simulink model "pulse_heating_official_spine_v04"  (R2025b)
settings: Solver=VariableStepAuto  StartTime=0.0  StopTime=0.25  RelTol=1e-3
PreLoadFcn:
  | addpath('C:\Users\ADMIN\Documents\MATLAB\Examples\R2025b\simscapeelectrical\BatteryThermalManagementExample');
  | addpath('C:\Users\ADMIN\Documents\MATLAB\Examples\R2025b\mcb\SIUnitsExample');
  | addpath('C:\Users\ADMIN\Documents\MATLAB\Examples\R2025b\simscapeelectrical\PMSMDriveThermalExample');
  | load_system('PMSMDriveThermal');
  | set_param('PMSMDriveThermal','SimscapeLogType','none','SimscapeLogSimulationStatistics','off');
  | set_param('PMSMDriveThermal','Dirty','off');
InitFcn:
  | % === M4-02A: Clean parameter matching (MO theory PI) ===
  | addpath('C:\Users\ADMIN\Documents\MATLAB\Examples\R2025b\simscapeelectrical\BatteryThermalManagementExample');
  | addpath('C:\Users\ADMIN\Documents\MATLAB\Examples\R2025b\mcb\SIUnitsExample');
  | addpath('C:\Users\ADMIN\Documents\MATLAB\Examples\R2025b\simscapeelectrical\PMSMDriveThermalExample');
  | load_system('PMSMDriveThermal');
  | PMSMDriveThermalData;
  | mcb_pmsm_foc_qep_f28379d_SIUnit_data;
  | clearvars('all');
  | 
  | % --- Construct clean pmsm struct from PMSMDriveThermal ---
  | pmsm = struct();
  | pmsm.Rs = Rs; pmsm.Ld = Ld; pmsm.Lq = Lq; pmsm.p = N; pmsm.FluxPM = PM;
  | pmsm.J = J; pmsm.B = 2.6369e-6; pmsm.I_rated = Imax;
  | pmsm.Ke = PM*N; pmsm.Kt = 1.5*N*PM; pmsm.N_max = 60*fnom/N;
  | pmsm.PositionOffset = 0; pmsm.QEPSlits = 1000;
  | 
  | inverter.V_dc = 70; dataType = 'double';
  | pmsm.N_base = inverter.V_dc / (sqrt(3)*PM*N*2*pi/60);
  | pmsm.T_rated = 1.5*N*PM*Imax;
  | 
  | % --- Timing (PMSMDriveThermal semantics) ---
  | Ts = 2e-6; fsw = 2e3; fc = fsw*10; Tsc = 1/fc;
  | T_pwm = 1/fsw; PWM_frequency = fsw; Ts_simulink = Tsc;
  | Ts_motor = Tsc; Ts_speed = 10*Tsc; Ts_inverter = Tsc;
  | 
  | % --- PI gains via mcb.calcFOCGains (MO theory) ---
  | motor = pmsm; motor.Rs = pmsm.Rs + inverter.R_board;
  | PI_params = mcb.calcFOCGains(motor, Tsc, Ts_speed, SpdLPFltCoeff=0.01);
  | PI_params.delay_Currents = int32(1);
  | PI_params.delay_Position = int32(1);
  | 
  | BatteryThermalManagementInitialization;
  | ambient = 263.15; coolantTemp = 263.15;
  | cellT_ini = ambient*ones(1,Ns*Np); cellT_ini4 = ambient*ones(1,Ns4*Np4);
  | Ns_total = 3*Ns + Ns4; Np_total = Np;
  | R_pack = Ns_total * R0_mat(3,2) / Np_total;
  | I_base_A = AH * Np_total; V_pack_nom = Ns_total * 3.3;
  | 
  | % === M4-01 generalized Reference / Platform contract ===
  | % Values are traceable engineering/platform defaults, not device ratings.
  | ReferenceConfig_ID = 'M4-01-REF-PLATFORM-v02';
  | ReferenceConfig_Source = 'OFFICIAL+ENGINEERING_DEFAULT';
  | ReferenceConfig_Scope = 'generalized_system_integration';
  | HVPath_R = 0.01;
  | DCLink_C = 470e-6;
  | DCLink_V0 = 0;
  | RMS_Window_s = 20/fsw;
  | IGBT_Ron_ref = 1e-3;
  | IGBT_Vf_ref = 1.2;
  | 
  | % Encoder/reference topology provides the static mechanical boundary.
  | OpenLoop_Vabc_Scale = 1;
model workspace (MAT data in the model file):
  control_status_v4d2_partial_duty_code = 6
  diagnostic_frequency_Hz = 50
  drive_status_v4d2_partial_current_code = 6
  kpi_status_v4d2_partial_numeric_code = 6
  kpi_value_unknown = nan
  limit_factor_unknown_code = 99
  limit_margin_unknown_value = nan
  limit_status_v4c_code = 5
  pulse_command_status_code = 6
  pulse_duty_percent = 50
  pulse_id_amplitude_A = 40
  pulse_iq_amplitude_A = 0
  pulse_mode_code = 4
  pulse_phase_delay_s = 0
undefined symbols (not defined in the file or in its folder): DiscIntNeverNeededParam, f_losses, Flowrate_vec, Isc_losses, losses_oc, losses_sc, N, PM, Rs
libraries: fl_lib x38, nesl_utility x35, ee_lib x12, mcbcontrolslib x5, mcbeeMathTransformLib x3, slpidlib x2, mcbhdlpositiondecoderlib x1, eePwmGeneratorTwoLevel x1
(part 4 of 4)

== system pulse_heating_official_spine_v04/PMSMDriveThermal_Inverter_And_Motor/Thermal model/Sensing Temperature WiA ==
  PS-Simulink Converter : nesl_utility/PS-Simulink Converter  PhysicalDomain=network_engine_domain  SubClassName=ps_output  LeftPortType=input  RightPortType=output  PseudoPeriodic=off  Frequencies=[]  VectorFormat=1-D array  Unit=degC  AffineConversion=on
  Temperature Sensor : fl_lib/Thermal/Thermal Sensors/Temperature Sensor  temperature_measure=foundation.enum.MeasurementReference.difference
  ThRef : fl_lib/Thermal/Thermal Elements/Thermal Reference
  H : PMIOPort  Side=Left
  tag scope: TA=global
  wires:
  PS-Simulink Converter/1 -> [TA]
  connections:
  Temperature Sensor/RConn2 -- PS-Simulink Converter/LConn1
  ThRef/LConn1 -- Temperature Sensor/RConn1
  H/RConn1 -- Temperature Sensor/LConn1

== system pulse_heating_official_spine_v04/PMSMDriveThermal_Inverter_And_Motor/Thermal model/Sensing Temperature WiB ==
  PS-Simulink Converter : nesl_utility/PS-Simulink Converter  PhysicalDomain=network_engine_domain  SubClassName=ps_output  LeftPortType=input  RightPortType=output  PseudoPeriodic=off  Frequencies=[]  VectorFormat=1-D array  Unit=degC  AffineConversion=on
  Temperature Sensor : fl_lib/Thermal/Thermal Sensors/Temperature Sensor  temperature_measure=foundation.enum.MeasurementReference.difference
  ThRef : fl_lib/Thermal/Thermal Elements/Thermal Reference
  H : PMIOPort  Side=Left
  tag scope: TB=global
  wires:
  PS-Simulink Converter/1 -> [TB]
  connections:
  H/RConn1 -- Temperature Sensor/LConn1
  ThRef/LConn1 -- Temperature Sensor/RConn1
  Temperature Sensor/RConn2 -- PS-Simulink Converter/LConn1

== system pulse_heating_official_spine_v04/PMSMDriveThermal_Inverter_And_Motor/Thermal model/Sensing Temperature WiC ==
  PS-Simulink Converter : nesl_utility/PS-Simulink Converter  PhysicalDomain=network_engine_domain  SubClassName=ps_output  LeftPortType=input  RightPortType=output  PseudoPeriodic=off  Frequencies=[]  VectorFormat=1-D array  Unit=degC  AffineConversion=on
  Temperature Sensor : fl_lib/Thermal/Thermal Sensors/Temperature Sensor  temperature_measure=foundation.enum.MeasurementReference.difference
  ThRef : fl_lib/Thermal/Thermal Elements/Thermal Reference
  H : PMIOPort  Side=Left
  tag scope: TC=global
  wires:
  PS-Simulink Converter/1 -> [TC]
  connections:
  Temperature Sensor/RConn2 -- PS-Simulink Converter/LConn1
  ThRef/LConn1 -- Temperature Sensor/RConn1
  H/RConn1 -- Temperature Sensor/LConn1

== system pulse_heating_official_spine_v04/BatteryThermalManagement_BatteryPack/Coolant_control/FlwR estimation/FlwR=f(cell_deltaT) ==
  Pack max T : Inport
  Pack min T : Inport  Port=2
  limit FlwR : Inport  Port=3
  MinMax4 : MinMax  Inputs=2  ZeroCross=off
  Multiply : Gain  Gain=0.1
  Subtract : Sum  Inputs=+-
  FlwR : Outport
  wires:
  Pack min T/1 -> Subtract/2
  MinMax4/1 -> FlwR/1
  Pack max T/1 -> Subtract/1
  Multiply/1 -> MinMax4/1
  limit FlwR/1 -> MinMax4/2
  Subtract/1 -> Multiply/1

== system pulse_heating_official_spine_v04/BatteryThermalManagement_BatteryPack/Coolant_control/FlwR estimation/FlwR=f(packT-ambientT) ==
  Pack max T : Inport
  FlwR limit : Inport  Port=2
  Ambient T : Inport  Port=3
  MinMax1 : MinMax  Inputs=2  ZeroCross=off
  Multiply1 : Gain  Gain=0.1
  Subtract1 : Sum  Inputs=+-
  FlwR : Outport
  wires:
  Ambient T/1 -> Subtract1/2
  MinMax1/1 -> FlwR/1
  Pack max T/1 -> Subtract1/1
  FlwR limit/1 -> MinMax1/1
  Multiply1/1 -> MinMax1/2
  Subtract1/1 -> Multiply1/1

== system pulse_heating_official_spine_v04/BatteryThermalManagement_BatteryPack/Coolant_control/Subsystem1/Flowrate-value ==
  FlwR : Inport
  Flowrate vector : Inport  Port=2
  MinMax6 : MinMax  Function=max  ZeroCross=off
  Product : Product
  Flowrate : Outport
  wires:
  Flowrate vector/1 -> MinMax6/1
  Product/1 -> Flowrate/1
  FlwR/1 -> Product/1
  MinMax6/1 -> Product/2

== system pulse_heating_official_spine_v04/BatteryThermalManagement_BatteryPack/Coolant_control/Subsystem1/FlwR limits ==
  FlwR : Inport
  MinMax5 : MinMax  Function=max  Inputs=2  ZeroCross=off
  MinMax7 : MinMax  Inputs=2  ZeroCross=off
  max value : Constant
  min value : Constant  Value=0.001
  FlwR_out : Outport
  wires:
  MinMax7/1 -> FlwR_out/1
  MinMax5/1 -> MinMax7/2
  FlwR/1 -> MinMax5/1
  max value/1 -> MinMax7/1
  min value/1 -> MinMax5/2

== system pulse_heating_official_spine_v04/BatteryThermalManagement_BatteryPack/Coolant_control/Subsystem1/Step generator ==
  frac : Inport
  step size : Inport  Port=2
  Max5 : MinMax  Function=max  Inputs=2  ZeroCross=off
  Minus4 : Sum  Inputs=+-
  Mod : Math  Operator=mod
  step output : Outport
  wires:
  frac/1 -> Mod/1, Minus4/1
  Max5/1 -> step output/1
  step size/1 -> Mod/2, Max5/2
  Mod/1 -> Minus4/2
  Minus4/1 -> Max5/1

== system pulse_heating_official_spine_v04/MCB_SIUnits_FOC_Controller/Control_System/Closed Loop Control/Current_Controllers ==
  Id : Inport
  Iq : Inport  Port=2
  Ida_ref : Inport  Port=3
  DQ Limiter : mcbcontrolslib/DQ Limiter  satMethodInputType=Specify via dialog  satMethodSelected=D-Q equivalence  satLimitInputType=Specify via dialog  Vmax=inverter.V_dc/sqrt(3) *0.95
  Demux : Demux  Outputs=2
  Mux : Mux
  PI_Controller_Id : Subsystem
  PI_Controller_Iq : Subsystem
  Terminator : Terminator
  Vd_ref : Outport  VectorParamsAs1DForOutWhenUnconnected=off
  Vq_ref : Outport  Port=2  VectorParamsAs1DForOutWhenUnconnected=off
  Idq : Outport  Port=3  VectorParamsAs1DForOutWhenUnconnected=off
  wires:
  DQ Limiter/3 -> Terminator/1
  DQ Limiter/1 -> Vd_ref/1
  DQ Limiter/2 -> Vq_ref/1
  PI_Controller_Iq/1(V_ref) -> DQ Limiter/2
  PI_Controller_Id/1(V_ref) -> DQ Limiter/1
  Mux/1 -> Idq/1
  Ida_ref/1 -> Demux/1
  Demux/2 -> PI_Controller_Iq/1(I_ref), Mux/3  "Iq_Ref"
  Demux/1 -> PI_Controller_Id/1(I_ref), Mux/1  "Id_Ref"
  Id/1 -> PI_Controller_Id/2(I_fb), Mux/2  "Id_fb"
  Iq/1 -> PI_Controller_Iq/2(I_fb), Mux/4  "Iq_fb"

== system pulse_heating_official_spine_v04/MCB_SIUnits_FOC_Controller/Control_System/Closed Loop Control/SVPWM ==
  Va : Inport
  Vb : Inport  Port=2
  Constant : Constant  Value=0.5  OutDataTypeStr=dataType  SampleTime=-1
  Mux1 : Mux  Inputs=3
  Normalize [-0.5 to 0.5] : Gain  Gain=1/ (2 * inverter.V_dc / sqrt(3))  RndMeth=Simplest  OutDataTypeStr=Inherit: Same as input
  Space Vector Generator : mcbcontrolslib/PWM Reference Generator  inSignal=Valphabeta  modType=SVM: space vector modulation
  Sum : Sum  Inputs=|++
  Duty_abc : Outport
  wires:
  Sum/1 -> Duty_abc/1
  Vb/1 -> Space Vector Generator/2
  Space Vector Generator/2 -> Mux1/2
  Space Vector Generator/3 -> Mux1/3
  Constant/1 -> Sum/2
  Space Vector Generator/1 -> Mux1/1
  Va/1 -> Space Vector Generator/1
  Normalize [-0.5 to 0.5]/1 -> Sum/1
  Mux1/1 -> Normalize [-0.5 to 0.5]/1

== system pulse_heating_official_spine_v04/MCB_SIUnits_FOC_Controller/Control_System/Open Loop Start-Up/Convert to Duty Cycles ==
  In : Inport
  Constant : Constant  Value=0.5  OutDataTypeStr=dataType  SampleTime=-1
  Normalize : Gain  Gain=1/2  RndMeth=Simplest  OutDataTypeStr=Inherit: Same as input
  Sum1 : Sum  Inputs=|++
  Out : Outport
  wires:
  Sum1/1 -> Out/1
  In/1 -> Normalize/1
  Constant/1 -> Sum1/2
  Normalize/1 -> Sum1/1

== system pulse_heating_official_spine_v04/MCB_SIUnits_FOC_Controller/Control_System/Open Loop Start-Up/Ramp Generator ==
  Ramp_Time : Inport
  Enable : Inport  Port=2
  Divide : Product  Inputs=*/  RndMeth=Simplest  OutDataTypeStr=Inherit: Same as first input
  NOT : Logic  Operator=NOT  IconShape=distinctive  AllPortsSameDT=off  OutDataTypeStr=boolean
  One : Constant  OutDataTypeStr=dataType  SampleTime=-1
  Ramp Generator : DiscreteIntegrator  IntegratorMethod=Accumulation: Forward Euler  gainval=1  ExternalReset=sampled level  SampleTime=-1  OutDataTypeStr=dataType  RndMeth=Simplest  LimitOutput=on  UpperSaturationLimit=1  LowerSaturationLimit=0  ICPrevOutput=DiscIntNeverNeededParam  ICPrevScaledInput=DiscIntNeverNeededParam
  Sample_Time : Gain  Gain=Tsc  RndMeth=Simplest  OutDataTypeStr=Inherit: Same as input
  Ramp : Outport
  wires:
  NOT/1 -> Ramp Generator/2
  Enable/1 -> NOT/1
  Ramp_Time/1 -> Divide/2
  One/1 -> Divide/1
  Sample_Time/1 -> Ramp Generator/1
  Ramp Generator/1 -> Ramp/1  "Eps"
  Divide/1 -> Sample_Time/1

== system pulse_heating_official_spine_v04/MCB_SIUnits_FOC_Controller/Control_System/Closed Loop Control/Current_Controllers/PI_Controller_Id ==
  I_ref : Inport
  I_fb : Inport  Port=2
  Data Store Read1 : DataStoreRead  DataStoreName=Enable  IndexOptions=Index vector (dialog)  Indices=1  OutputSizes=1
  Discrete PI Controller with anti-windup & reset : slpidlib/PID Controller  Controller=PI  Form=Parallel  TimeDomain=Discrete-time  UseExternalTs=off  SampleTime=-1  IntegratorMethod=Forward Euler  FilterMethod=Forward Euler  ControllerParametersSource=external  P=1  I=1  UseKiTs=on  D=0  UseExternalDerivativeSource=off  N=100  UseFilter=on  TunerSelectOption=Transfer Function Based (PID Tuner App)  InitialConditionSource=external  InitialConditionForIntegrator=0  InitialConditionForFilter=0  DifferentiatorICPrevScaledInput=0  ExternalReset=level  TrackingMode=off  Kt=1  LimitOutput=on  SatLimitsSource=internal  UpperSaturationLimit=inverter.V_dc/sqrt(3)  LowerSaturationLimit=-inverter.V_dc/sqrt(3)  LinearizeAsGain=on  AntiWindupMode=clamping  Kb=1  LimitIntegrator=off  UpperIntegratorSaturationLimit=inf  LowerIntegratorSaturationLimit=-inf  RndMeth=Simplest  POutMin=[]  POutMax=[]  IOutMin=[]  IOutMax=[]  DOutMin=[]  DOutMax=[]  NOutMin=[]  NOutMax=[]  SumOutMin=[]  SumOutMax=[]  SaturationOutDataTypeStr=Inherit: Inherit via back propagation  SaturationOutMin=[]  SaturationOutMax=[]  PParamMin=[]  PParamMax=[]  IParamMin=[]  IParamMax=[]  DParamMin=[]  DParamMax=[]  NParamMin=[]  NParamMax=[]  KbParamMin=[]  KbParamMax=[]  KtParamMin=[]  KtParamMax=[]  KbOutMin=[]  KbOutMax=[]  KtOutMin=[]  KtOutMax=[]  IntegratorOutMin=[]  IntegratorOutMax=[]  FilterOutMin=[]  FilterOutMax=[]  SumI1OutMin=[]  SumI1OutMax=[]  SumI2OutMin=[]  SumI2OutMax=[]  SumI3OutMin=[]  SumI3OutMax=[]  SumI4OutMin=[]  SumI4OutMax=[]  SumDOutMin=[]  SumDOutMax=[]  DifferentiatorOutMin=[]  DifferentiatorOutMax=[]  FilterDiffOutCoefMin=[]  FilterDiffOutCoefMax=[]  ReciprocalOutMin=[]  ReciprocalOutMax=[]  SumDenOutMin=[]  SumDenOutMax=[]  SumNumOutMin=[]  SumNumOutMax=[]  DivideOutMin=[]  DivideOutMax=[]  UdiffTsProdOutMin=[]  UdiffTsProdOutMax=[]  NTsProdOutMin=[]  NTsProdOutMax=[]  UintegralTsProdOutMin=[]  UintegralTsProdOutMax=[]  UngainTsProdOutMin=[]  UngainTsProdOutMax=[]  ClampingZeroOutDataTypeStr=Inherit: Inherit via back propagation  ClampingZeroOutMin=[]  ClampingZeroOutMax=[]  FilterDenConstantOutDataTypeStr=Inherit: Inherit via back propagation  FilterDenConstantOutMin=[]  FilterDenConstantOutMax=[]  PCopyOutDataTypeStr=Inherit: Inherit via back propagation  PCopyOutMin=[]  PCopyOutMax=[]  NCopyOutDataTypeStr=Inherit: Inherit via back propagation  NCopyOutMin=[]  NCopyOutMax=[]  IntegratorContinuousStateAttributes=''  IntegratorStateMustResolveToSignalObject=off  IntegratorRTWStateStorageClass=Auto  FilterContinuousStateAttributes=''  FilterStateMustResolveToSignalObject=off  FilterRTWStateStorageClass=Auto  ParallelPVariant=ExternalParameters  IdealPVariant=Disabled  IVariant=ExternalParameters  DVariant=Disabled  IntegratorVariant=Discrete  SatVariant=Enabled  AWVariant=DiscClampingParallel  PCopyVariant=Disabled  TRVariant=Disabled  FdbkBlocksVariant=Forward  IdealPFdbkVariant=Disabled  SatFdbkVariant=Disabled  DerivativeFilterVariant=Disabled  NVariant=Disabled  NCopyVariant=Disabled_SignalSpec  FilterICVariant=Disabled  IntegratorICVariant=ExternalICs  ExternalResetVariant=ExternalReset  TRSumVariant=Passthrough  SumFdbkVariant=Disabled  SumVariant=Sum_PI  TsampFilterVariant=InternalTs  TsampNgainVariant=Passthrough  TsampIntegralVariant=Disabled_SignalSpec  ExternalSaturationOutDataTypeStr=Inherit: Same as second input  DerivativeSourceVariant=Disabled  PreIntVariant=InternalPreInt
      settings: LibrarySourceBlock=mcbcontrolslib/PI Controller
  Ki : Constant  Value=PI_params.Ki_i * Tsc  OutDataTypeStr=dataType  SampleTime=-1
  Ki1 : Constant  Value=0  OutDataTypeStr=dataType  SampleTime=-1
  Kp : Constant  Value=PI_params.Kp_i  OutDataTypeStr=dataType  SampleTime=-1
  Logical Operator : Logic  Operator=NOT  IconShape=distinctive  AllPortsSameDT=off  OutDataTypeStr=boolean
  Sum : Sum  Inputs=|+-  OutDataTypeStr=Inherit: Same as first input
  V_ref : Outport  VectorParamsAs1DForOutWhenUnconnected=off
  wires:
  Ki1/1 -> Discrete PI Controller with anti-windup & reset/5
  Logical Operator/1 -> Discrete PI Controller with anti-windup & reset/4
  Ki/1 -> Discrete PI Controller with anti-windup & reset/3
  Kp/1 -> Discrete PI Controller with anti-windup & reset/2
  Sum/1 -> Discrete PI Controller with anti-windup & reset/1
  Discrete PI Controller with anti-windup & reset/1 -> V_ref/1
  Data Store Read1/1 -> Logical Operator/1
  I_fb/1 -> Sum/2
  I_ref/1 -> Sum/1

== system pulse_heating_official_spine_v04/MCB_SIUnits_FOC_Controller/Control_System/Closed Loop Control/Current_Controllers/PI_Controller_Iq ==
  I_ref : Inport
  I_fb : Inport  Port=2
  Data Store Read1 : DataStoreRead  DataStoreName=Enable  IndexOptions=Index vector (dialog)  Indices=1  OutputSizes=1
  Discrete PI Controller with anti-windup & reset : slpidlib/PID Controller  Controller=PI  Form=Parallel  TimeDomain=Discrete-time  UseExternalTs=off  SampleTime=-1  IntegratorMethod=Forward Euler  FilterMethod=Forward Euler  ControllerParametersSource=external  P=1  I=1  UseKiTs=on  D=0  UseExternalDerivativeSource=off  N=100  UseFilter=on  TunerSelectOption=Transfer Function Based (PID Tuner App)  InitialConditionSource=external  InitialConditionForIntegrator=0  InitialConditionForFilter=0  DifferentiatorICPrevScaledInput=0  ExternalReset=level  TrackingMode=off  Kt=1  LimitOutput=on  SatLimitsSource=internal  UpperSaturationLimit=inverter.V_dc/sqrt(3)  LowerSaturationLimit=-inverter.V_dc/sqrt(3)  LinearizeAsGain=on  AntiWindupMode=clamping  Kb=1  LimitIntegrator=off  UpperIntegratorSaturationLimit=inf  LowerIntegratorSaturationLimit=-inf  RndMeth=Simplest  POutMin=[]  POutMax=[]  IOutMin=[]  IOutMax=[]  DOutMin=[]  DOutMax=[]  NOutMin=[]  NOutMax=[]  SumOutMin=[]  SumOutMax=[]  SaturationOutDataTypeStr=Inherit: Inherit via back propagation  SaturationOutMin=[]  SaturationOutMax=[]  PParamMin=[]  PParamMax=[]  IParamMin=[]  IParamMax=[]  DParamMin=[]  DParamMax=[]  NParamMin=[]  NParamMax=[]  KbParamMin=[]  KbParamMax=[]  KtParamMin=[]  KtParamMax=[]  KbOutMin=[]  KbOutMax=[]  KtOutMin=[]  KtOutMax=[]  IntegratorOutMin=[]  IntegratorOutMax=[]  FilterOutMin=[]  FilterOutMax=[]  SumI1OutMin=[]  SumI1OutMax=[]  SumI2OutMin=[]  SumI2OutMax=[]  SumI3OutMin=[]  SumI3OutMax=[]  SumI4OutMin=[]  SumI4OutMax=[]  SumDOutMin=[]  SumDOutMax=[]  DifferentiatorOutMin=[]  DifferentiatorOutMax=[]  FilterDiffOutCoefMin=[]  FilterDiffOutCoefMax=[]  ReciprocalOutMin=[]  ReciprocalOutMax=[]  SumDenOutMin=[]  SumDenOutMax=[]  SumNumOutMin=[]  SumNumOutMax=[]  DivideOutMin=[]  DivideOutMax=[]  UdiffTsProdOutMin=[]  UdiffTsProdOutMax=[]  NTsProdOutMin=[]  NTsProdOutMax=[]  UintegralTsProdOutMin=[]  UintegralTsProdOutMax=[]  UngainTsProdOutMin=[]  UngainTsProdOutMax=[]  ClampingZeroOutDataTypeStr=Inherit: Inherit via back propagation  ClampingZeroOutMin=[]  ClampingZeroOutMax=[]  FilterDenConstantOutDataTypeStr=Inherit: Inherit via back propagation  FilterDenConstantOutMin=[]  FilterDenConstantOutMax=[]  PCopyOutDataTypeStr=Inherit: Inherit via back propagation  PCopyOutMin=[]  PCopyOutMax=[]  NCopyOutDataTypeStr=Inherit: Inherit via back propagation  NCopyOutMin=[]  NCopyOutMax=[]  IntegratorContinuousStateAttributes=''  IntegratorStateMustResolveToSignalObject=off  IntegratorRTWStateStorageClass=Auto  FilterContinuousStateAttributes=''  FilterStateMustResolveToSignalObject=off  FilterRTWStateStorageClass=Auto  ParallelPVariant=ExternalParameters  IdealPVariant=Disabled  IVariant=ExternalParameters  DVariant=Disabled  IntegratorVariant=Discrete  SatVariant=Enabled  AWVariant=DiscClampingParallel  PCopyVariant=Disabled  TRVariant=Disabled  FdbkBlocksVariant=Forward  IdealPFdbkVariant=Disabled  SatFdbkVariant=Disabled  DerivativeFilterVariant=Disabled  NVariant=Disabled  NCopyVariant=Disabled_SignalSpec  FilterICVariant=Disabled  IntegratorICVariant=ExternalICs  ExternalResetVariant=ExternalReset  TRSumVariant=Passthrough  SumFdbkVariant=Disabled  SumVariant=Sum_PI  TsampFilterVariant=InternalTs  TsampNgainVariant=Passthrough  TsampIntegralVariant=Disabled_SignalSpec  ExternalSaturationOutDataTypeStr=Inherit: Same as second input  DerivativeSourceVariant=Disabled  PreIntVariant=InternalPreInt
      settings: LibrarySourceBlock=mcbcontrolslib/PI Controller
  Ki : Constant  Value=PI_params.Ki_i * Tsc  OutDataTypeStr=dataType  SampleTime=-1
  Kp : Constant  Value=PI_params.Kp_i  OutDataTypeStr=dataType  SampleTime=-1
  Kp1 : Constant  Value=0  OutDataTypeStr=dataType  SampleTime=-1
  Logical Operator : Logic  Operator=NOT  IconShape=distinctive  AllPortsSameDT=off  OutDataTypeStr=boolean
  Sum : Sum  Inputs=|+-  OutDataTypeStr=Inherit: Same as first input
  V_ref : Outport  VectorParamsAs1DForOutWhenUnconnected=off
  wires:
  Kp1/1 -> Discrete PI Controller with anti-windup & reset/5
  Logical Operator/1 -> Discrete PI Controller with anti-windup & reset/4
  Ki/1 -> Discrete PI Controller with anti-windup & reset/3
  Sum/1 -> Discrete PI Controller with anti-windup & reset/1
  Kp/1 -> Discrete PI Controller with anti-windup & reset/2
  I_ref/1 -> Sum/1
  I_fb/1 -> Sum/2
  Data Store Read1/1 -> Logical Operator/1
  Discrete PI Controller with anti-windup & reset/1 -> V_ref/1

== matlab function pulse_heating_official_spine_v04/System_Audit/Energy_And_Thermal_Audit/Energy_Balance_Audit ==
  settings: updateMethod=DISCRETE  sampleTime=1e-3
  data: V_pack input; P_batt_terminal output; I_pack input; P_cu input; P_iron input; P_inv input; P_batt_heat input; w_motor input; trq_motor input; P_loss_total output; residual_dc_link output; P_charge output; P_discharge output; V_dc input; I_dc input; P_hv_loss_in input; DeltaE_dc_link_in input; P_thermal_storage_in input; P_heat_rejection_in input; P_dc_input output; P_hv_loss output; DeltaE_dc_link output; P_thermal_storage output; P_unmodeled output; ledger_valid output; P_loss_known output; P_mech output; P_heat_rejection output; P_dc_link_storage_in input; E_dc_link_in input; Q_hv_gen_in input; P_dc_link_storage output; E_dc_link output; Q_hv_gen output; DeltaE_batt_in input; DeltaE_batt output
function [P_batt_terminal, P_loss_total, residual_dc_link, P_charge, P_discharge, P_dc_input, P_hv_loss, DeltaE_dc_link, P_thermal_storage, P_unmodeled, ledger_valid, P_loss_known, P_mech, P_heat_rejection, P_dc_link_storage, E_dc_link, Q_hv_gen, DeltaE_batt] = fcn(V_pack, I_pack, P_cu, P_iron, P_inv, P_batt_heat, w_motor, trq_motor, V_dc, I_dc, P_hv_loss_in, DeltaE_dc_link_in, P_thermal_storage_in, P_heat_rejection_in, P_dc_link_storage_in, E_dc_link_in, Q_hv_gen_in, DeltaE_batt_in)
% E5+G4: unknown-aware ledger with explicit DC-link, battery-storage, and thermal fields.
% Positive battery terminal power denotes discharge under the existing V4 sign convention.
% P_dc_link_storage is d(E_dc_link)/dt in W; E_dc_link, DeltaE_dc_link, and DeltaE_batt are reporting-window fields in J.
% P_unmodeled and residual_dc_link are the signed DC-boundary mismatch, not external assumed values.
% Thermal storage and heat rejection remain independent reporting fields to avoid double counting.
P_batt_terminal = V_pack * I_pack;
P_mech = w_motor * trq_motor;
P_loss_known = P_inv + P_cu + P_iron + P_batt_heat;
P_dc_input = V_dc * I_dc;
P_hv_loss = P_hv_loss_in;
P_dc_link_storage = P_dc_link_storage_in;
E_dc_link = E_dc_link_in;
DeltaE_dc_link = DeltaE_dc_link_in;
DeltaE_batt = DeltaE_batt_in;
P_thermal_storage = P_thermal_storage_in;
P_heat_rejection = P_heat_rejection_in;
Q_hv_gen = Q_hv_gen_in;
valid_batt = ~(isnan(P_batt_terminal) || isinf(P_batt_terminal));
valid_dc = ~(isnan(P_dc_input) || isinf(P_dc_input));
valid_known_loss = ~(isnan(P_loss_known) || isinf(P_loss_known));
valid_hv = ~(isnan(P_hv_loss_in) || isinf(P_hv_loss_in));
valid_dc_storage = ~(isnan(P_dc_link_storage_in) || isinf(P_dc_link_storage_in));
valid_edc = ~(isnan(E_dc_link_in) || isinf(E_dc_link_in));
valid_delta_e = ~(isnan(DeltaE_dc_link_in) || isinf(DeltaE_dc_link_in));
valid_delta_batt = ~(isnan(DeltaE_batt_in) || isinf(DeltaE_batt_in));
valid_thermal = ~(isnan(P_thermal_storage_in) || isinf(P_thermal_storage_in)) && ~(isnan(P_heat_rejection_in) || isinf(P_heat_rejection_in));
valid_qhv = ~(isnan(Q_hv_gen_in) || isinf(Q_hv_gen_in));
if valid_known_loss && valid_hv
    P_loss_total = P_loss_known + P_hv_loss_in;
else
    P_loss_total = NaN;
end
if valid_batt && valid_dc && valid_hv && valid_dc_storage
    residual_dc_link = P_batt_terminal - P_hv_loss_in - P_dc_link_storage_in - P_dc_input;
    P_unmodeled = residual_dc_link;
else
    residual_dc_link = NaN;
    P_unmodeled = NaN;
end
if I_pack >= 0 && valid_batt
    P_discharge = P_batt_terminal;
    P_charge = 0;
elseif valid_batt
    P_discharge = 0;
    P_charge = -P_batt_terminal;
else
    P_discharge = NaN;
    P_charge = NaN;
end
ledger_valid = double(valid_batt && valid_dc && valid_known_loss && valid_hv && valid_dc_storage && valid_edc && valid_delta_e && valid_delta_batt && valid_thermal && valid_qhv);
end

== matlab function pulse_heating_official_spine_v04/System_Audit/RMS_And_Measurement_Audit/Compute_I_rms_V4G ==
  settings: updateMethod=DISCRETE  sampleTime=1e-3
  data: I_batt input; I_batt_rms output; I_dc input; i_phase input; I_heat_equiv input; t input; window_s input; I_dc_rms output; I_phase_rms output; I_heat_equiv_rms output; window_complete output; window_elapsed_s output
function [I_batt_rms, I_dc_rms, I_phase_rms, I_heat_equiv_rms, window_complete, window_elapsed_s] = fcn(I_batt, I_dc, i_phase, I_heat_equiv, t, window_s)
% G2: time-window RMS for distinct electrical and thermal-equivalent channels
% The integral uses actual Clock time increments and trapezoidal mean-square accumulation.
% Outputs remain NaN until a complete valid window is available.
% I_heat_equiv is intentionally separate and remains invalid until a defined producer exists.
persistent initialized t_prev window_start batt_sq dc_sq phase_sq heat_sq
persistent batt_prev dc_prev phase_prev heat_prev batt_valid dc_valid phase_valid heat_valid
persistent last_batt last_dc last_phase last_heat last_window_s has_result
I_batt_rms = NaN;
I_dc_rms = NaN;
I_phase_rms = NaN;
I_heat_equiv_rms = NaN;
window_complete = 0;
window_elapsed_s = NaN;
if isnan(window_s) || isinf(window_s) || window_s <= 0
    return;
end
current_batt_valid = ~(isnan(I_batt) || isinf(I_batt));
current_dc_valid = ~(isnan(I_dc) || isinf(I_dc));
current_phase_valid = ~any(isnan(i_phase)) && ~any(isinf(i_phase));
current_heat_valid = ~(isnan(I_heat_equiv) || isinf(I_heat_equiv));
if isempty(initialized)
    initialized = true;
    t_prev = t;
    window_start = t;
    batt_sq = 0;
    dc_sq = 0;
    phase_sq = 0;
    heat_sq = 0;
    batt_prev = I_batt;
    dc_prev = I_dc;
    phase_prev = i_phase;
    heat_prev = I_heat_equiv;
    batt_valid = current_batt_valid;
    dc_valid = current_dc_valid;
    phase_valid = current_phase_valid;
    heat_valid = current_heat_valid;
    last_batt = NaN;
    last_dc = NaN;
    last_phase = NaN;
    last_heat = NaN;
    last_window_s = NaN;
    has_result = false;
    return;
end
dt = t - t_prev;
if isnan(dt) || isinf(dt) || dt <= 0
    t_prev = t;
    return;
end
if batt_valid && current_batt_valid
    batt_sq = batt_sq + 0.5 * dt * (batt_prev^2 + I_batt^2);
else
    batt_valid = false;
end
if dc_valid && current_dc_valid
    dc_sq = dc_sq + 0.5 * dt * (dc_prev^2 + I_dc^2);
else
    dc_valid = false;
end
phase_prev_sq = sum(phase_prev.^2) / numel(phase_prev);
phase_now_sq = sum(i_phase.^2) / numel(i_phase);
if phase_valid && current_phase_valid
    phase_sq = phase_sq + 0.5 * dt * (phase_prev_sq + phase_now_sq);
else
    phase_valid = false;
end
if heat_valid && current_heat_valid
    heat_sq = heat_sq + 0.5 * dt * (heat_prev^2 + I_heat_equiv^2);
else
    heat_valid = false;
end
t_prev = t;
batt_prev = I_batt;
dc_prev = I_dc;
phase_prev = i_phase;
heat_prev = I_heat_equiv;
window_elapsed = t - window_start;
if window_elapsed >= window_s
    if batt_valid
        last_batt = sqrt(batt_sq / window_elapsed);
    else
        last_batt = NaN;
    end
    if dc_valid
        last_dc = sqrt(dc_sq / window_elapsed);
    else
        last_dc = NaN;
    end
    if phase_valid
        last_phase = sqrt(phase_sq / window_elapsed);
    else
        last_phase = NaN;
    end
    if heat_valid
        last_heat = sqrt(heat_sq / window_elapsed);
    else
        last_heat = NaN;
    end
    has_result = true;
    last_window_s = window_elapsed;
    window_complete = 1;
    window_start = t;
    batt_sq = 0;
    dc_sq = 0;
    phase_sq = 0;
    heat_sq = 0;
    batt_valid = current_batt_valid;
    dc_valid = current_dc_valid;
    phase_valid = current_phase_valid;
    heat_valid = current_heat_valid;
end
if has_result
    I_batt_rms = last_batt;
    I_dc_rms = last_dc;
    I_phase_rms = last_phase;
    I_heat_equiv_rms = last_heat;
end
end

== matlab function pulse_heating_official_spine_v04/KPI_And_Logging/Compute_Voltage_Margin_V4G ==
  data: V_dc input; V_margin output; mod_index input
function V_margin = fcn(V_dc, mod_index)
% G3: Voltage margin = V_dc * (1 - modulation_index)
% mod_index from ControlKPI[2] = max(abs(2*duty_abc - 1))
% V_margin > 0 means voltage headroom available
% V_margin <= 0 means over-modulation (saturation)
V_margin = V_dc * (1 - mod_index);
end

== matlab function pulse_heating_official_spine_v04/BatteryThermalManagement_BatteryPack/Compute_T_min_V4F ==
  data: Pack_T input; T_min output
function T_min = fcn(Pack_T)
% F1: Minimum pack temperature from 4 module temperatures
% Pack_T = [T_module1; T_module2; T_module3; T_module4]
T_min = min(Pack_T);
end

== matlab function pulse_heating_official_spine_v04/System_Audit/Battery_Envelope_Screening/Compute_Battery_Limits_V4F ==
  data: T_min input; charge_limit output; SOC input; cellAH input; discharge_limit output
function [charge_limit, discharge_limit] = fcn(T_min, SOC, cellAH)
% F3: Battery charge/discharge current limits based on temperature and SOC
% I_base = cellAH (loaded as I_base_A = AH*Np = 40A from InitFcn)
% Charge: T>=0C full; T<0C derated by f(T)*g(SOC)
% Discharge: T>=-10C full; T<-10C derated 50%
I_base = cellAH;

if T_min >= 273.15
    f_T = 1.0;
else
    f_T = max(0.1, (T_min - 253.15) / 20.0);
end

if SOC >= 0.8
    g_SOC = max(0.1, (1.0 - SOC) / 0.2);
else
    g_SOC = 1.0;
end

charge_limit = I_base * f_T * g_SOC;

if T_min < 263.15
    discharge_limit = I_base * 0.5;
else
    discharge_limit = I_base;
end
end

== matlab function pulse_heating_official_spine_v04/System_Audit/Battery_Envelope_Screening/Compute_Lithium_Risk_V4F ==
  data: T_min input; risk_flag output; I_pack input; charge_limit input; safety_margin output
function [risk_flag, safety_margin] = fcn(T_min, I_pack, charge_limit)
% F5: Lithium plating risk proxy (PLACEHOLDER - not safety conclusion)
% risk_flag: 0=safe, 1=warning, 2=risk
T_charge_cutoff = 273.15;
I_abs = abs(I_pack);
safety_margin = charge_limit - I_abs;

if T_min < T_charge_cutoff && I_abs > charge_limit
    risk_flag = 2;
elseif T_min < T_charge_cutoff && safety_margin < charge_limit * 0.2
    risk_flag = 1;
else
    risk_flag = 0;
end
end

== matlab function pulse_heating_official_spine_v04/BatteryThermalManagement_BatteryPack/Sel_SOC_min_V4F ==
  data: SOC_limits input; SOC_min output
function SOC_min = fcn(SOC_limits)
% F2: Extract SOC_min from [SOC_min; SOC_max] vector
SOC_min = SOC_limits(1);
end

== matlab function pulse_heating_official_spine_v04/MCB_SIUnits_FOC_Controller/Control_System/Closed Loop Control/Inverse_Clarke_Vabc ==
  data: Valpha input; Vabc output; Vbeta input
function Vabc = fcn(Valpha, Vbeta)
% Inverse Clarke: alpha-beta to abc
Va = Valpha;
Vb = -0.5*Valpha + sqrt(3)/2*Vbeta;
Vc = -0.5*Valpha - sqrt(3)/2*Vbeta;
Vabc = [Va; Vb; Vc];
end

== matlab function pulse_heating_official_spine_v04/System_Audit/Energy_And_Thermal_Audit/Compute_P_cu_V4E ==
  data: Idq_debug input; P_cu output; Rs input
function P_cu = fcn(Idq_debug, Rs)
% E1: Motor copper loss P_cu = 1.5 * Rs * (Id^2 + Iq^2)
Id_fb = Idq_debug(2);
Iq_fb = Idq_debug(4);
P_cu = 1.5 * Rs * (Id_fb^2 + Iq_fb^2);
end

== matlab function pulse_heating_official_spine_v04/PMSMDriveThermal_Inverter_And_Motor/Scopes/losses/MATLAB Function ==
  data: i_d input; trq_loss output; i_q input; w input; PM parameter; N parameter; losses_oc parameter; losses_sc parameter; f_losses parameter; Isc_losses parameter
function trq_loss = fcn(i_d,i_q,w,PM, N, losses_oc, losses_sc, f_losses, Isc_losses)

lambda = 2*pi*PM/(sqrt(2)*N);
a_h = losses_oc(1)/f_losses;
a_J = losses_oc(2)/f_losses^2;
a_ex = losses_oc(3)/f_losses^1.5;

b_h = losses_sc(1)/f_losses;
b_J = losses_sc(2)/f_losses^2;
b_ex = losses_sc(3)/f_losses^1.5;

Id = abs(i_d)/sqrt(2);
w_abs = abs(w);
if Id>0.999*Isc_losses
    ratio_Id_Isc = 0.999;
else
    ratio_Id_Isc = Id/Isc_losses;
end
Vd = lambda*w_abs*N/(2*pi)*ratio_Id_Isc; 
Iq = abs(i_q)/sqrt(2);
Vm = lambda*w_abs*N/(2*pi)*sqrt((1-ratio_Id_Isc)^2+(Iq/Isc_losses)^2);

Vm_losses = a_h/lambda*Vm+a_J/lambda^2*Vm^2+a_ex/lambda^1.5*Vm^1.5;
Vd_losses = b_h/lambda*Vd+b_J/lambda^2*Vd^2+b_ex/lambda^1.5*Vd^1.5;

trq_loss = sign(w)*(Vd_losses+Vm_losses)/(w_abs+1);

== matlab function pulse_heating_official_spine_v04/PMSMDriveThermal_Inverter_And_Motor/Compute_Current_KPI_V4D2 ==
  data: i_abc input; i_rms output; i_peak output
function [i_rms, i_peak] = f(i_abc)
                                  i = i_abc(:);                      
                                  i_rms = sqrt(sum(i.^2)/numel(i));  
                                  i_peak = max(abs(i));              
                                  end

== matlab function pulse_heating_official_spine_v04/MCB_SIUnits_FOC_Controller/Compute_Duty_KPI_V4D2 ==
  data: duty_abc input; mod_index output; sat_flag output
function [mod_index, sat_flag] = f(duty_abc)
                                           d = duty_abc(:);                            
                                           mod_index = max(abs(2*d - 1));              
                                           sat_flag = double(any(d <= 0 | d >= 1));    
                                           end

== matlab function pulse_heating_official_spine_v04/System_Audit/Energy_And_Thermal_Audit/Compute_P_iron_V4E ==
  data: trq_loss input; P_iron output; w_motor input
function P_iron = fcn(trq_loss, w_motor)
% E2: Motor iron loss P_iron = trq_loss * w_motor
% At stall (w~0), P_iron ~ 0
P_iron = abs(trq_loss .* w_motor);
end

== matlab function pulse_heating_official_spine_v04/System_Audit/Energy_And_Thermal_Audit/Compute_P_inv_V4E ==
  data: i_abc input; P_inv output; Ron input; Vf input
function P_inv = fcn(i_abc, Ron, Vf)
% E3: Inverter conduction loss (2 IGBTs conduct at any time)
% P_cond = 2*(Vf*I_avg + Ron*I_rms^2)
i = i_abc(:);
I_rms = sqrt(sum(i.^2)/numel(i));
I_avg = mean(abs(i));
P_inv = 2 * (Vf * I_avg + Ron * I_rms^2);
end

== matlab function pulse_heating_official_spine_v04/System_Audit/Energy_And_Thermal_Audit/Compute_P_batt_heat_V4E ==
  data: I_pack input; P_batt_heat output; R_pack input
function P_batt_heat = fcn(I_pack, R_pack)
% E4: Battery heat generation P = I^2 * R_pack
% R_pack = Ns_total * R0_cell / Np (from InitFcn, OFFICIAL source)
P_batt_heat = I_pack^2 * R_pack;
end
